simulink model "simTest02"  (R2020b)
settings: Solver=VariableStepAuto  StartTime=0.0  StopTime=10.0  RelTol=1e-3
model workspace (MAT data in the model file):
  K = Simulink.Parameter
  K.Value = [1 1 1]
  K.DataType = 'auto'
  K.Dimensions = [1 3]
  th = Simulink.Parameter
  th.DataType = 'auto'
  th.Dimensions = [0 0]
  v = Simulink.Parameter
  v.DataType = 'auto'
  v.Dimensions = [0 0]
  veri01 = [0  1  0  0; 0  0  1  0; 0  0  0  1; -1  0  -2  0]
settings Model: Creator=GM-ROBOT  LastModifiedBy=root

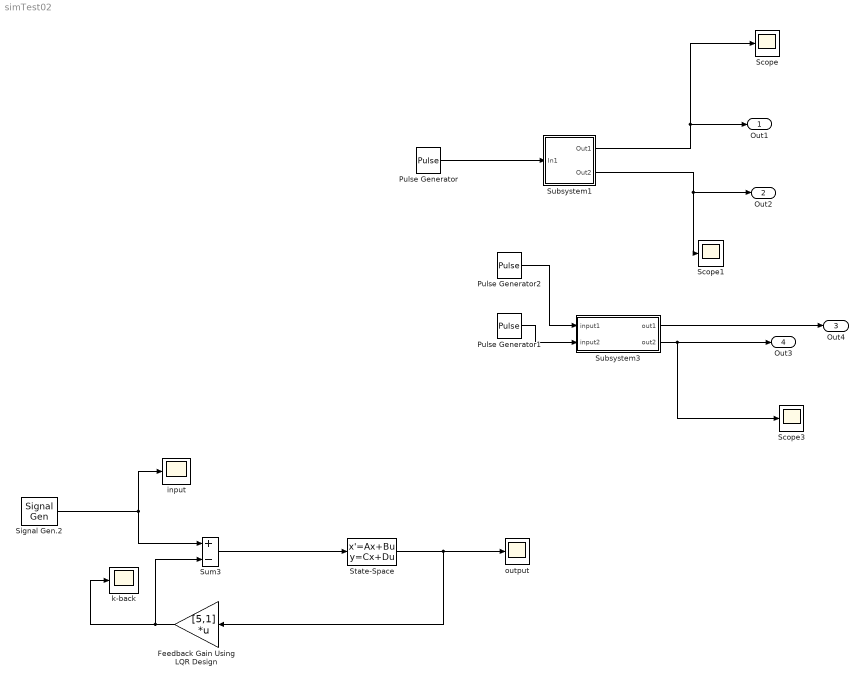
== system simTest02 ==
  Feedback Gain Using LQR Design : Gain  Gain=[5,1]  Multiplication=Matrix(K*u) (u vector)
  Pulse Generator : DiscretePulseGenerator  PulseType=Time based  Period=10  PulseWidth=5
  Pulse Generator1 : DiscretePulseGenerator  PulseType=Time based  Period=10  PulseWidth=5
  Pulse Generator2 : DiscretePulseGenerator  PulseType=Time based  Period=10  PulseWidth=5
  Scope : Scope
  Scope1 : Scope
  Scope3 : Scope
  Signal Gen.2 : SignalGenerator  Amplitude=2
  State-Space : StateSpace  A=[1,1;2,2]  B=[1;1]  C=[2,2;3,3]  D=[1;1]  InitialCondition=0
  Subsystem1 : Subsystem
  Subsystem3 : Subsystem  mask{gain1=2, gain2=3, Parameter3=0}
  Sum3 : Sum  Inputs=+-  InputSameDT=on  SaturateOnIntegerOverflow=on  OutDataTypeStr=Inherit: Same as first input
  input : Scope
  k-back : Scope
  output : Scope
  Out1 : Outport
  Out2 : Outport  Port=2
  Out4 : Outport  Port=3
  Out3 : Outport  Port=4
  wires:
  Subsystem1/1(Out1) -> Scope/1, Out1/1
  Subsystem1/2(Out2) -> Scope1/1, Out2/1
  Pulse Generator/1 -> Subsystem1/1(In1)
  Pulse Generator1/1 -> Subsystem3/2("input2 ")
  Pulse Generator2/1 -> Subsystem3/1(input1)
  Subsystem3/1(out1) -> Out4/1
  Subsystem3/2(out2) -> Scope3/1, Out3/1
  Signal Gen.2/1 -> Sum3/1, input/1
  Feedback Gain Using LQR Design/1 -> k-back/1, Sum3/2
  Sum3/1 -> State-Space/1
  State-Space/1 -> output/1, Feedback Gain Using LQR Design/1

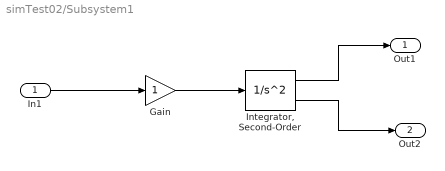
== system simTest02/Subsystem1 ==
  In1 : Inport
  Gain : Gain
  "Integrator, Second-Order" : SecondOrderIntegrator
  Out1 : Outport
  Out2 : Outport  Port=2
  wires:
  Gain/1 -> "Integrator, Second-Order"/1
  "Integrator, Second-Order"/1 -> Out1/1
  "Integrator, Second-Order"/2 -> Out2/1
  In1/1 -> Gain/1

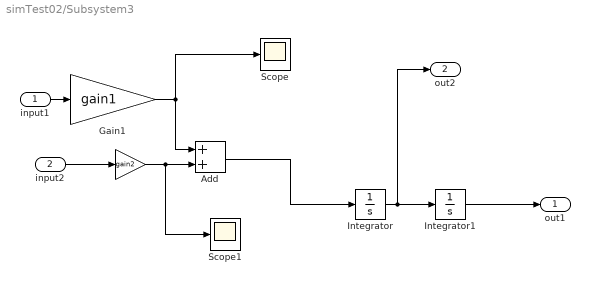
== system simTest02/Subsystem3 ==
  input1 : Inport
  "input2 " : Inport  Port=2
  " " : Gain  Gain=gain2
  Add : Sum
  Gain1 : Gain  Gain=gain1
  Integrator : Integrator
  Integrator1 : Integrator
  Scope : Scope
  Scope1 : Scope
  out1 : Outport
  out2 : Outport  Port=2
  wires:
  Gain1/1 -> Add/1, Scope/1
  input1/1 -> Gain1/1
  Integrator/1 -> out2/1, Integrator1/1
  "input2 "/1 -> " "/1
  Add/1 -> Integrator/1
  Integrator1/1 -> out1/1
  " "/1 -> Scope1/1, Add/2
